simulink model "bloczki_1"  (R2015a)
settings: Solver=ode45  StartTime=0.0  StopTime=10.0  RelTol=1e-3
libraries: simulink x2
settings Model: Creator=Jaromir  LastModifiedBy=Jaromir

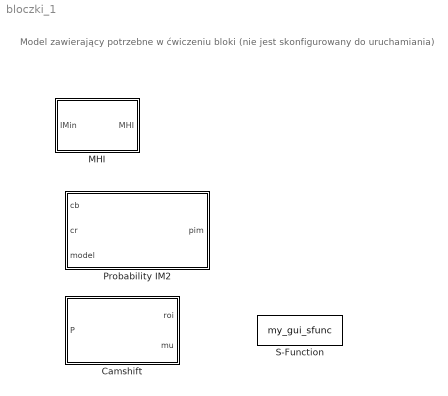
== system bloczki_1 ==
  note: Model zawierający potrzebne w ćwiczeniu bloki (nie jest skonfigurowany do uruchamiania)
  Camshift : MATLAB Function  TreatAsAtomicUnit=on
  MHI : Subsystem  mask{tres=12, Tau=6}
      mask prompts: tres "Motion treshold"; Tau "Tau parameter"
  Probability IM2 : MATLAB Function  TreatAsAtomicUnit=on
  S-Function : S-Function  FunctionName=my_gui_sfunc

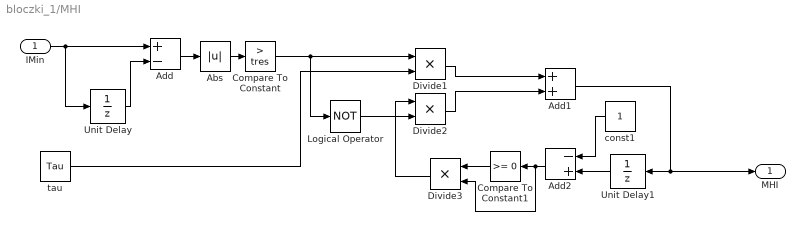
== system bloczki_1/MHI ==
  IMin : Inport
  Abs : Abs
  Add : Sum  Inputs=+-  OutDataTypeStr=int16
  Add1 : Sum  OutDataTypeStr=double
  Add2 : Sum  Inputs=-+  OutDataTypeStr=double
  Compare To Constant : simulink/Logic and Bit Operations/Compare To Constant  relop=>  const=tres  OutDataTypeStr=uint8  ZeroCross=off
  Compare To Constant1 : simulink/Logic and Bit Operations/Compare To Constant  relop=>=  const=0  OutDataTypeStr=uint8  ZeroCross=off
  Divide1 : Product  Inputs=**
  Divide2 : Product  Inputs=**
  Divide3 : Product  Inputs=**
  Logical Operator : Logic  Operator=NOT  AllPortsSameDT=off  OutDataTypeStr=boolean
  Unit Delay : UnitDelay  SampleTime=-1
  Unit Delay1 : UnitDelay  SampleTime=-1
  const1 : Constant
  tau : Constant  Value=Tau
  MHI : Outport
  wires:
  Unit Delay/1 -> Add/2
  Add/1 -> Abs/1
  Abs/1 -> Compare To Constant/1
  tau/1 -> Divide1/2
  Logical Operator/1 -> Divide2/2
  Divide1/1 -> Add1/1
  Divide2/1 -> Add1/2
  Add1/1 -> Unit Delay1/1, MHI/1
  Unit Delay1/1 -> Add2/2
  const1/1 -> Add2/1
  Add2/1 -> Compare To Constant1/1, Divide3/2
  Compare To Constant1/1 -> Divide3/1
  Divide3/1 -> Divide2/1
  IMin/1 -> Add/1, Unit Delay/1
  Compare To Constant/1 -> Logical Operator/1, Divide1/1

== matlab function bloczki_1/Probability IM2 ==
  data: cb input; cr input; model input; pim output
function pim = probabilityIM2(cb,cr,model)
%#codegen
% Wyznaczenie tablicy prawdopodobienstwa dla obrazu wg zadanego modelu koloru skory.
%
% INPUT:
% > im - testowy obraz wejsciowy w formacie RGB
% > model - model koloru skory (tablica [256*256])
% OUTPUT:                                                                         
% > skin_model - obraz prawdopodobienstwa
%
% DEPENDICIES:
% -
% COMMENTS:
% > Wykorzystano przeksztalcenie look-up-table 2D
% > TODO kontrola argumentow wejsciowych
% CREATED: Jaromir Przybylo, 26.10.2015, R2015a
% LASTMODIFIED: 
%

ind=sub2ind([256 256],cb(:),cr(:));
outim=model(ind);
pim=reshape(outim,size(cb(:,:,1)));

== matlab function bloczki_1/Camshift ==
  data: P input; roi output; mu output
function [roi,mu]=Camshift(P)
%#codegen
% Uproszczony algorytm CAMSHIFT
%
% INPUT:
% > P       - obraz prawdopodobienstwa <0-1>
% OUTPUT:                                                                         
% > roi     - wspolrzedne ROI sledzonego obiektu [x,y,w,h]
% > mu      - wspolrzedne srodka ROI [x,y]
%
% DEPENDICIES:
% -
% COMMENTS:
% > TODO kontrola argumentow wejsciowych oraz optymalizacja kodu pod
%   wzgledem szybkosci
% CREATED: Jaromir Przybylo, 26.10.2015, R2015a
% LASTMODIFIED: 
%

% Inicjalizacja
S = -100;
Sp = 100;
[m,n]=size(P);
[mm,nn]=meshgrid(1:n,1:m);
P1=double(P);
BW=ones(m,n);
mm1=mm;nn1=nn;
roi  = uint32([1 1 m n]);
MU=uint32([m/2 n/2]);

% Camshift (bardzo uproszczony)
while abs(S-Sp)>1
    Sp=S;
    P1=P.*BW;
    mm1=mm.*BW;
    nn1=nn.*BW;
    
    m00=sum(sum(P1));
    m10=sum(sum(P1.*mm1));
    m01=sum(sum(P1.*nn1));
    
    MU=uint32([m10/m00 m01/m00]);
    S=2*sqrt(1*m00/1);
    
    min1=max([round(MU-S/2);1 1]);
    max1=min([round(MU+S/2);n m]);
    
    roi  = uint32([MU(1)-S/2 MU(2)-S/2 S S]);
    
    BW=zeros(m,n);
    BW(min1(2):max1(2),min1(1):max1(1))=1;    
end      

roi=roi;
mu=MU;
